simulink library "DQN_Machines"  (R2023b)
settings: Solver=VariableStepAuto  StartTime=0.0  StopTime=10.0  RelTol=1e-3
undefined symbols (not defined in the file): DiscIntNeverNeededParam, N, SM, Ts
libraries: spsabctodq0Lib x2, spsdq0toabcLib x2
(part 4 of 5)

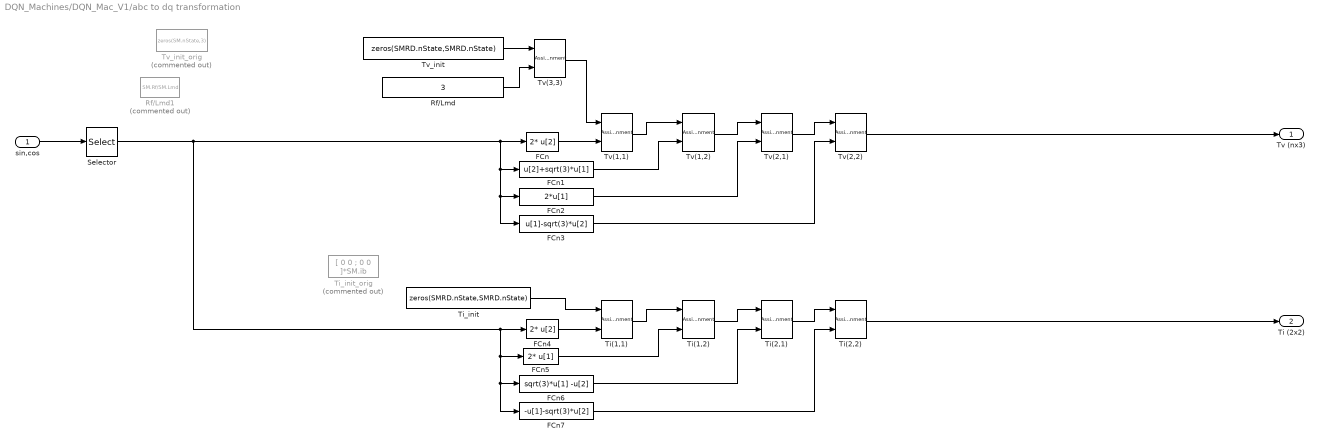
== system DQN_Machines/DQN_Mac_V1/abc to dq transformation ==
  sin,cos : Inport
  FCn : Fcn  Expr=2* u[2]  SampleTime=Ts
  FCn1 : Fcn  Expr=u[2]+sqrt(3)*u[1]  SampleTime=Ts
  FCn2 : Fcn  Expr=2*u[1]  SampleTime=Ts
  FCn3 : Fcn  Expr=u[1]-sqrt(3)*u[2]  SampleTime=Ts
  FCn4 : Fcn  Expr=2* u[2]  SampleTime=Ts
  FCn5 : Fcn  Expr=2* u[1]  SampleTime=Ts
  FCn6 : Fcn  Expr=sqrt(3)*u[1] -u[2]  SampleTime=Ts
  FCn7 : Fcn  Expr=-u[1]-sqrt(3)*u[2]  SampleTime=Ts
  Rf/Lmd : Constant  Value=3
  Rf/Lmd1 : Constant  Commented=on  Value=SM.Rf/SM.Lmd
  Selector : Selector  InputPortWidth=2  IndexOptions=Index vector (dialog)  Indices=[1 2]  OutputSizes=1
  "Ti(1,1) " : Assignment  NumberOfDimensions=2  DiagnosticForDimensions=Warning  IndexOptions=Index vector (dialog),Index vector (dialog)  Indices=1,1  OutputSizes=1,1
  "Ti(1,2) " : Assignment  NumberOfDimensions=2  DiagnosticForDimensions=Warning  IndexOptions=Index vector (dialog),Index vector (dialog)  Indices=1,2  OutputSizes=1,1
  "Ti(2,1) " : Assignment  NumberOfDimensions=2  DiagnosticForDimensions=Warning  IndexOptions=Index vector (dialog),Index vector (dialog)  Indices=2,1  OutputSizes=1,1
  "Ti(2,2) " : Assignment  NumberOfDimensions=2  DiagnosticForDimensions=Warning  IndexOptions=Index vector (dialog),Index vector (dialog)  Indices=2,2  OutputSizes=1,1
  Ti_init : Constant  Value=zeros(SMRD.nState,SMRD.nState)
  Ti_init_orig : Constant  Commented=on  Value="[ 0  0 ;  0  0  ]*SM.ib"
  Tv(1,1) : Assignment  NumberOfDimensions=2  DiagnosticForDimensions=Warning  IndexOptions=Index vector (dialog),Index vector (dialog)  Indices=1,1  OutputSizes=1,1
  Tv(1,2) : Assignment  NumberOfDimensions=2  DiagnosticForDimensions=Warning  IndexOptions=Index vector (dialog),Index vector (dialog)  Indices=1,2  OutputSizes=1,1
  Tv(2,1) : Assignment  NumberOfDimensions=2  DiagnosticForDimensions=Warning  IndexOptions=Index vector (dialog),Index vector (dialog)  Indices=2,1  OutputSizes=1,1
  Tv(2,2) : Assignment  NumberOfDimensions=2  DiagnosticForDimensions=Warning  IndexOptions=Index vector (dialog),Index vector (dialog)  Indices=2,2  OutputSizes=1,1
  Tv(3,3) : Assignment  NumberOfDimensions=2  DiagnosticForDimensions=Warning  IndexOptions=Index vector (dialog),Index vector (dialog)  Indices=3,3  OutputSizes=1,1
  Tv_init : Constant  Value=zeros(SMRD.nState,SMRD.nState)
  Tv_init_orig : Constant  Commented=on  Value=zeros(SM.nState,3)
  Tv (nx3) : Outport  VectorParamsAs1DForOutWhenUnconnected=off
  Ti (2x2) : Outport  Port=2  VectorParamsAs1DForOutWhenUnconnected=off
  wires:
  Tv(3,3)/1 -> Tv(1,1)/1
  Rf/Lmd/1 -> Tv(3,3)/2
  Tv_init/1 -> Tv(3,3)/1
  FCn7/1 -> "Ti(2,2) "/2
  "Ti(2,1) "/1 -> "Ti(2,2) "/1
  "Ti(1,2) "/1 -> "Ti(2,1) "/1
  FCn6/1 -> "Ti(2,1) "/2
  FCn5/1 -> "Ti(1,2) "/2
  "Ti(1,1) "/1 -> "Ti(1,2) "/1
  FCn4/1 -> "Ti(1,1) "/2
  FCn3/1 -> Tv(2,2)/2
  Tv(2,1)/1 -> Tv(2,2)/1
  Tv(1,2)/1 -> Tv(2,1)/1
  FCn2/1 -> Tv(2,1)/2
  FCn1/1 -> Tv(1,2)/2
  Tv(1,1)/1 -> Tv(1,2)/1
  FCn/1 -> Tv(1,1)/2
  sin,cos/1 -> Selector/1
  Ti_init/1 -> "Ti(1,1) "/1
  Selector/1 -> FCn7/1, FCn6/1, FCn5/1, FCn4/1, FCn/1, FCn1/1, FCn2/1, FCn3/1
  Tv(2,2)/1 -> Tv (nx3)/1
  "Ti(2,2) "/1 -> Ti (2x2)/1

== system DQN_Machines/DQN_Mac_V1/sin,cos ==
  theta : Inport
  Elementary Math : Trigonometry
  Elementary Math1 : Trigonometry  Operator=cos
  Mux3 : Mux  Inputs=2
  sin,cos : Outport  InitialOutput=0  VectorParamsAs1DForOutWhenUnconnected=off
  wires:
  theta/1 -> Elementary Math/1, Elementary Math1/1
  Elementary Math/1 -> Mux3/1
  Elementary Math1/1 -> Mux3/2
  Mux3/1 -> sin,cos/1

== system DQN_Machines/#BACKUP/DQN_Mac_V1/Discretize BE or Tustin2 ==
  note: Implement discretized state-space model using Tustin or TBE method
      |
      | BE      -> SM.DSSmethod=1
      | Tustin  -> SM.DSSmethod=2
      |
      |
      | Tustin
      | ------
      | Ad = inv(I - Ts/2*A)*(I + Ts/2*A)
      | Bd = inv(I - Ts/2*A)*B
      | Cd = C*inv(I - Ts/2*A)*Ts
      | Dd = C*inv(I - Ts/2*A)*B*Ts/2  + D  =  Cd*B/2
      |
      | TBE
      | ---
      | Ad = inv(I - Ts*A)
      | Bd = inv(I - Ts*A)*B
      | Cd = C*inv(I - Ts*A)*Ts
      | Dd = C*inv(I - Ts*A)*B*Ts  + D  =  Cd*B
      |
      | I = eye(SM.nState,SM.nState)
  A : Inport
  B : Inport  Port=2
  C : Inport  Port=3
  I : Constant  Value=eye(SMRD.nState,SMRD.nState)
  Product{1..4} (4 alike) : Product  Multiplication=Matrix(*)  SaturateOnIntegerOverflow=on  OutDataTypeStr=Inherit: Same as first input
  Sum1 : Sum  Inputs=+-  SaturateOnIntegerOverflow=on
  Sum5 : Sum  SaturateOnIntegerOverflow=on
  "Tustin: 1/2 BE : 1.0" : Gain  Gain=0.5  SaturateOnIntegerOverflow=on  OutDataTypeStr=Inherit: Same as input  ParamDataTypeStr=Inherit: Same as input
  "Tustin: Ts/2 BE : Ts" : Gain  Gain=SMRD.Ts/2  SaturateOnIntegerOverflow=on  OutDataTypeStr=Inherit: Same as input  ParamDataTypeStr=Inherit: Same as input
  inversion : Product  Inputs=/  Multiplication=Matrix(*)  RndMeth=Zero
  wbase3 : Gain  Gain=Ts  SaturateOnIntegerOverflow=on  OutDataTypeStr=Inherit: Same as input  ParamDataTypeStr=Inherit: Same as input
  Ad : Outport  VectorParamsAs1DForOutWhenUnconnected=off
  Bd : Outport  Port=2  VectorParamsAs1DForOutWhenUnconnected=off
  Cd : Outport  Port=3  VectorParamsAs1DForOutWhenUnconnected=off
  Dd : Outport  Port=4  VectorParamsAs1DForOutWhenUnconnected=off
  inv(I_Ts/2*A) : Outport  Port=5  VectorParamsAs1DForOutWhenUnconnected=off
  wires:
  "Tustin: Ts/2 BE : Ts"/1 -> Sum1/2, Sum5/2
  Product4/1 -> Ad/1
  A/1 -> "Tustin: Ts/2 BE : Ts"/1
  I/1 -> Sum5/1, Sum1/1
  Sum1/1 -> inversion/1
  inversion/1 -> Product2/2, Product1/1, Product4/1, inv(I_Ts/2*A)/1
  Sum5/1 -> Product4/2
  Product1/1 -> Bd/1
  B/1 -> Product1/2, Product3/2
  C/1 -> Product2/1
  Product2/1 -> wbase3/1
  Product3/1 -> "Tustin: 1/2 BE : 1.0"/1
  "Tustin: 1/2 BE : 1.0"/1 -> Dd/1
  wbase3/1 -> Cd/1, Product3/1

== system DQN_Machines/#BACKUP/DQN_Mac_V1/Electromagnetic Torque2 ==
  note: Te computed from stator fluxes and currents
  note: Te=phids*Iqs - phiqs*Ids
  phiqd : Inport
  iqd : Inport  Port=2
  1-1 : Gain  Gain=[-1 1]
  Mult1 : Product  Inputs=**
  Selector1 : Selector  InputPortWidth=2  IndexOptions=Index vector (dialog)  Indices="[2  1]"  OutputSizes=1
  Sum2 : Sum  Inputs=1  SaturateOnIntegerOverflow=on
  Te : Outport  VectorParamsAs1DForOutWhenUnconnected=off
  wires:
  phiqd/1 -> Selector1/1
  Mult1/1 -> Sum2/1
  iqd/1 -> 1-1/1
  1-1/1 -> Mult1/2  "iqs -ids"
  Selector1/1 -> Mult1/1  "phids phiqs"
  Sum2/1 -> Te/1

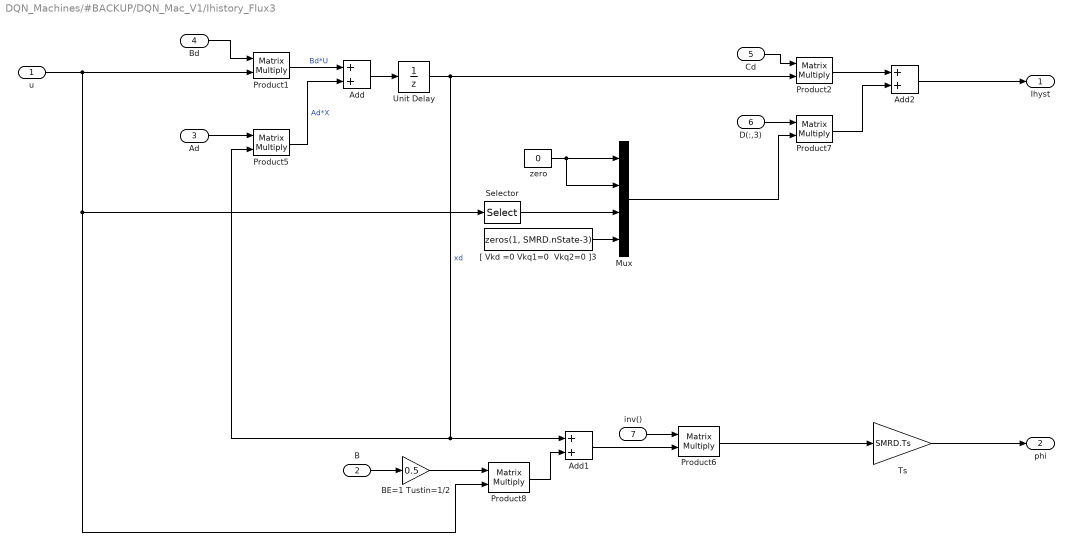
== system DQN_Machines/#BACKUP/DQN_Mac_V1/Ihistory_Flux3 ==
  u : Inport
  B : Inport  Port=2
  Ad : Inport  Port=3
  Bd : Inport  Port=4
  Cd : Inport  Port=5
  D(:,3) : Inport  Port=6
  inv() : Inport  Port=7
  Add : Sum
  Add1 : Sum
  Add2 : Sum
  BE=1 Tustin=1/2 : Gain  Gain=0.5
  Mux : Mux
  Product{1..2,5..8} (6 alike) : Product  Multiplication=Matrix(*)  SaturateOnIntegerOverflow=on  OutDataTypeStr=Inherit: Same as first input
  Selector : Selector  InputPortWidth=SMRD.nState  IndexOptions=Index vector (dialog)  Indices=[3]  OutputSizes=1
  Ts : Gain  Gain=SMRD.Ts  SaturateOnIntegerOverflow=on  OutDataTypeStr=Inherit: Same as input  ParamDataTypeStr=Inherit: Same as input
  Unit Delay : UnitDelay  InitialCondition=SMRD.phidq0(1:SMRD.nState)/SMRD.Ts  SampleTime=SMRD.Ts  HasFrameUpgradeWarning=on
  "[ Vkd =0 Vkq1=0  Vkq2=0 ]3" : Constant  Value=zeros(1, SMRD.nState-3)
  zero : Constant  Value=0
  Ihyst : Outport  VectorParamsAs1DForOutWhenUnconnected=off
  phi : Outport  Port=2  VectorParamsAs1DForOutWhenUnconnected=off
  wires:
  BE=1 Tustin=1/2/1 -> Product8/1
  u/1 -> Product1/2, Product8/2, Selector/1
  B/1 -> BE=1 Tustin=1/2/1
  inv()/1 -> Product6/1
  Cd/1 -> Product2/1
  Bd/1 -> Product1/1
  Ad/1 -> Product5/1
  Add1/1 -> Product6/2
  Product8/1 -> Add1/2
  Product6/1 -> Ts/1
  Product5/1 -> Add/2  "Ad*X"
  Unit Delay/1 -> Product5/2, Add1/1, Product2/2  "xd"
  Add/1 -> Unit Delay/1
  Product1/1 -> Add/1  "Bd*U"
  Ts/1 -> phi/1
  Product2/1 -> Add2/1
  Add2/1 -> Ihyst/1
  Mux/1 -> Product7/2
  D(:,3)/1 -> Product7/1
  "[ Vkd =0 Vkq1=0  Vkq2=0 ]3"/1 -> Mux/4
  zero/1 -> Mux/2, Mux/1
  Selector/1 -> Mux/3
  Product7/1 -> Add2/2

== system DQN_Machines/#BACKUP/DQN_Mac_V1/Matrix W3 ==
  wr : Inport
  Gain1 : Gain  Gain=-1  SaturateOnIntegerOverflow=on  OutDataTypeStr=Inherit: Same as input  ParamDataTypeStr=Inherit: Same as input
  Gain2 : Gain  Gain=-1  SaturateOnIntegerOverflow=on  OutDataTypeStr=Inherit: Same as input  ParamDataTypeStr=Inherit: Same as input
  W(1,2)=wr : Assignment  NumberOfDimensions=2  IndexOptions=Index vector (dialog),Index vector (dialog)  Indices=1,2  OutputSizes=1,1
  W(2,1)=-wr : Assignment  NumberOfDimensions=2  IndexOptions=Index vector (dialog),Index vector (dialog)  Indices=2,1  OutputSizes=1,1
  u1 : Constant  Value=zeros(SMRD.nState,SMRD.nState)
  "[W]" : Outport  VectorParamsAs1DForOutWhenUnconnected=off
  wires:
  u1/1 -> W(1,2)=wr/1
  Gain1/1 -> W(2,1)=-wr/2
  W(1,2)=wr/1 -> W(2,1)=-wr/1
  wr/1 -> W(1,2)=wr/2, Gain1/1
  W(2,1)=-wr/1 -> Gain2/1
  Gain2/1 -> "[W]"/1

== system DQN_Machines/#BACKUP/DQN_Mac_V1/Mechanical model ==
  note: *
  note: Computation of Rotor angle dthetae uses Forward Euler
      | integrator to ensure better accuracy and initialisation.
  note: *
  Te : Inport  PortDimensions=1
  Pm : Inport  Port=2
  1 ----- 2H : Gain  Gain=1/(2*SMRD.H)  SaturateOnIntegerOverflow=on  OutDataTypeStr=Inherit: Same as input  ParamDataTypeStr=Inherit: Same as input
  1_Pb : Gain  Gain=1/SMRD.Pb  SaturateOnIntegerOverflow=on  OutDataTypeStr=Inherit: Same as input  ParamDataTypeStr=Inherit: Same as input
  Delay Prediction : Subsystem
  Digital Clock : DigitalClock  SampleTime=Ts
  F : Gain  Gain=SMRD.F  SaturateOnIntegerOverflow=on  OutDataTypeStr=Inherit: Same as input  ParamDataTypeStr=Inherit: Same as input
  Mux1 : Mux  Inputs=2
  Rate Transition1 : RateTransition  Deterministic=off  OutPortSampleTime=Ts
  Rotor angle dthetae : DiscreteIntegrator  InitialCondition=SMRD.tho  SampleTime=SMRD.Ts  ICPrevOutput=DiscIntNeverNeededParam  ICPrevScaledInput=DiscIntNeverNeededParam
  Rotor speed deviation (dw) : DiscreteIntegrator  IntegratorMethod=Integration: Trapezoidal  InitialCondition=SMRD.dwo  SampleTime=SMRD.Ts  ICPrevOutput=DiscIntNeverNeededParam  ICPrevScaledInput=DiscIntNeverNeededParam
  Sum : Sum  InputSameDT=on  SaturateOnIntegerOverflow=on  OutDataTypeStr=Inherit: Same as first input
  Sum2 : Sum  Inputs=+--  InputSameDT=on  SaturateOnIntegerOverflow=on  OutDataTypeStr=Inherit: Same as first input
  Sum3 : Sum  InputSameDT=on  SaturateOnIntegerOverflow=on  OutDataTypeStr=Inherit: Same as first input
  div : Fcn  Expr=u[2]/u[1]
      mask Display: disp('/')
  nominal speed : Constant
  we base : Gain  Gain=SMRD.wn  SaturateOnIntegerOverflow=on  OutDataTypeStr=Inherit: Same as input  ParamDataTypeStr=Inherit: Same as input
  web2 : Gain  Gain=SMRD.wn  SaturateOnIntegerOverflow=on  OutDataTypeStr=Inherit: Same as input  ParamDataTypeStr=Inherit: Same as input
  dtheta_e : Outport  InitialOutput=0  VectorParamsAs1DForOutWhenUnconnected=off
  we : Outport  Port=2  InitialOutput=0  VectorParamsAs1DForOutWhenUnconnected=off
  theta_e : Outport  Port=3  InitialOutput=0  VectorParamsAs1DForOutWhenUnconnected=off
  wires:
  Delay Prediction/1(dw) -> we base/1, Sum/2  "dw"
  Rate Transition1/1 -> 1_Pb/1
  Rotor angle dthetae/1 -> Sum3/1, dtheta_e/1  "d_theta (rad)"
  web2/1 -> Sum3/2
  Digital Clock/1 -> web2/1
  we base/1 -> Rotor angle dthetae/1
  Rotor speed deviation (dw)/1 -> Delay Prediction/1(in)  "dw"
  nominal speed/1 -> Sum/1
  1 ----- 2H/1 -> Rotor speed deviation (dw)/1
  div/1 -> Sum2/1
  Te/1 -> Sum2/2  "Te"
  Mux1/1 -> div/1
  Pm/1 -> Rate Transition1/1  "Pm"
  1_Pb/1 -> Mux1/2
  F/1 -> Sum2/3
  Sum2/1 -> 1 ----- 2H/1
  Sum/1 -> F/1, we/1, Mux1/1  "n"
  Sum3/1 -> theta_e/1

== system DQN_Machines/#BACKUP/DQN_Mac_V1_old/Electromagnetic Torque1 ==
  note: Te computed from stator fluxes and currents
  note: Te=phids*Iqs - phiqs*Ids
  phiqd : Inport
  iqd : Inport  Port=2
  1-1 : Gain  Gain=[-1 1]
  Mult1 : Product  Inputs=**
  Selector1 : Selector  InputPortWidth=2  IndexOptions=Index vector (dialog)  Indices="[2  1]"  OutputSizes=1
  Sum2 : Sum  Inputs=1  SaturateOnIntegerOverflow=on
  Te : Outport  VectorParamsAs1DForOutWhenUnconnected=off
  wires:
  phiqd/1 -> Selector1/1
  Mult1/1 -> Sum2/1
  iqd/1 -> 1-1/1
  1-1/1 -> Mult1/2  "iqs -ids"
  Selector1/1 -> Mult1/1  "phids phiqs"
  Sum2/1 -> Te/1

== system DQN_Machines/#BACKUP/DQN_Mac_V1_old/Ihistory_Flux ==
  A : Inport
  u_dq : Inport  Port=2
  Add2 : Sum
  Add3 : Sum
  BE=1 Tustin=1/2 : Gain  Gain=0.5
  I : Constant  Value=eye(SMRD.nState,SMRD.nState)
  Product{4..5,7..8} (4 alike) : Product  Multiplication=Matrix(*)  SaturateOnIntegerOverflow=on  OutDataTypeStr=Inherit: Same as first input
  Sum1 : Sum  Inputs=+-  SaturateOnIntegerOverflow=on
  Sum5 : Sum  SaturateOnIntegerOverflow=on
  Ts : Gain  Gain=SMRD.Ts  SaturateOnIntegerOverflow=on  OutDataTypeStr=Inherit: Same as input  ParamDataTypeStr=Inherit: Same as input
  "Tustin: Ts/2 BE : Ts" : Gain  Gain=SMRD.Ts/2  SaturateOnIntegerOverflow=on  OutDataTypeStr=Inherit: Same as input  ParamDataTypeStr=Inherit: Same as input
  Unit Delay2 : UnitDelay  InitialCondition=SMRD.phidq0/SMRD.Ts  SampleTime=SMRD.Ts  HasFrameUpgradeWarning=on
  inversion : Product  Inputs=/  Multiplication=Matrix(*)  RndMeth=Zero
  phi : Outport  VectorParamsAs1DForOutWhenUnconnected=off
  wires:
  Unit Delay2/1 -> Add3/1, Product4/2  "xd"
  Add2/1 -> Unit Delay2/1
  Product4/1 -> Add2/2  "Ad*X"
  Product5/1 -> Product4/1
  Product7/1 -> Ts/1
  Add3/1 -> Product7/2
  inversion/1 -> Product7/1, Product8/1, Product5/1
  Ts/1 -> phi/1
  u_dq/1 -> Product8/2, BE=1 Tustin=1/2/1
  Sum1/1 -> inversion/1
  Sum5/1 -> Product5/2
  I/1 -> Sum5/1, Sum1/1
  A/1 -> "Tustin: Ts/2 BE : Ts"/1
  "Tustin: Ts/2 BE : Ts"/1 -> Sum5/2, Sum1/2
  BE=1 Tustin=1/2/1 -> Add3/2
  Product8/1 -> Add2/1

== system DQN_Machines/#BACKUP/DQN_Mac_V1_old/Matrix W3 ==
  wr : Inport
  Gain1 : Gain  Gain=-1  SaturateOnIntegerOverflow=on  OutDataTypeStr=Inherit: Same as input  ParamDataTypeStr=Inherit: Same as input
  W(1,2)=wr : Assignment  NumberOfDimensions=2  IndexOptions=Index vector (dialog),Index vector (dialog)  Indices=1,2  OutputSizes=1,1
  W(2,1)=-wr : Assignment  NumberOfDimensions=2  IndexOptions=Index vector (dialog),Index vector (dialog)  Indices=2,1  OutputSizes=1,1
  u1 : Constant  Value=zeros(SMRD.nState,SMRD.nState)
  "[W]" : Outport  VectorParamsAs1DForOutWhenUnconnected=off
  wires:
  u1/1 -> W(1,2)=wr/1
  wr/1 -> W(2,1)=-wr/2, W(1,2)=wr/2
  W(1,2)=wr/1 -> Gain1/1
  W(2,1)=-wr/1 -> "[W]"/1
  Gain1/1 -> W(2,1)=-wr/1

== system DQN_Machines/#BACKUP/DQN_Mac_V1_old/Mechanical model ==
  note: *
  note: Computation of Rotor angle dthetae uses Forward Euler
      | integrator to ensure better accuracy and initialisation.
  note: *
  Te : Inport  PortDimensions=1
  Pm : Inport  Port=2
  1 ----- 2H : Gain  Gain=1/(2*SMRD.H)  SaturateOnIntegerOverflow=on  OutDataTypeStr=Inherit: Same as input  ParamDataTypeStr=Inherit: Same as input
  1_Pb : Gain  Gain=1/SMRD.Pb  SaturateOnIntegerOverflow=on  OutDataTypeStr=Inherit: Same as input  ParamDataTypeStr=Inherit: Same as input
  Delay Prediction : Subsystem
  Digital Clock : DigitalClock  SampleTime=SMRD.Ts
  F : Gain  Gain=SMRD.F  SaturateOnIntegerOverflow=on  OutDataTypeStr=Inherit: Same as input  ParamDataTypeStr=Inherit: Same as input
  Mux1 : Mux  Inputs=2
  Rate Transition1 : RateTransition  Commented=on  Deterministic=off  OutPortSampleTime=SMRD.Ts
  Rotor angle dthetae : DiscreteIntegrator  InitialCondition=SMRD.tho  SampleTime=SMRD.Ts  ICPrevOutput=DiscIntNeverNeededParam  ICPrevScaledInput=DiscIntNeverNeededParam
  Rotor speed deviation (dw) : DiscreteIntegrator  IntegratorMethod=Integration: Trapezoidal  InitialCondition=SMRD.dwo  SampleTime=SMRD.Ts  ICPrevOutput=DiscIntNeverNeededParam  ICPrevScaledInput=DiscIntNeverNeededParam
  Sum : Sum  InputSameDT=on  SaturateOnIntegerOverflow=on  OutDataTypeStr=Inherit: Same as first input
  Sum2 : Sum  Inputs=+--  InputSameDT=on  SaturateOnIntegerOverflow=on  OutDataTypeStr=Inherit: Same as first input
  Sum3 : Sum  InputSameDT=on  SaturateOnIntegerOverflow=on  OutDataTypeStr=Inherit: Same as first input
  div : Fcn  Expr=u[2]/u[1]
      mask Display: disp('/')
  nominal speed : Constant
  we base : Gain  Gain=SMRD.web  SaturateOnIntegerOverflow=on  OutDataTypeStr=Inherit: Same as input  ParamDataTypeStr=Inherit: Same as input
  web2 : Gain  Gain=SMRD.web  SaturateOnIntegerOverflow=on  OutDataTypeStr=Inherit: Same as input  ParamDataTypeStr=Inherit: Same as input
  we : Outport
  theta_e : Outport  Port=2  InitialOutput=0  VectorParamsAs1DForOutWhenUnconnected=off
  dtheta_e : Outport  Port=3  InitialOutput=0  VectorParamsAs1DForOutWhenUnconnected=off
  wires:
  Delay Prediction/1(dw) -> we base/1, Sum/2  "dw"
  Rotor angle dthetae/1 -> dtheta_e/1, Sum3/1  "d_theta (rad)"
  web2/1 -> Sum3/2
  Digital Clock/1 -> web2/1
  we base/1 -> Rotor angle dthetae/1
  Rotor speed deviation (dw)/1 -> Delay Prediction/1(in)  "dw"
  nominal speed/1 -> Sum/1
  1 ----- 2H/1 -> Rotor speed deviation (dw)/1
  div/1 -> Sum2/1
  Te/1 -> Sum2/2  "Te"
  Mux1/1 -> div/1
  Pm/1 -> 1_Pb/1  "Pm"
  1_Pb/1 -> Mux1/2
  F/1 -> Sum2/3
  Sum2/1 -> 1 ----- 2H/1
  Sum/1 -> F/1, we/1, Mux1/1  "n"
  Sum3/1 -> theta_e/1

== system DQN_Machines/#BACKUP/DQN_Mac_V1_old/mac_pnz2dq_conv ==
  In1 : Inport
  Complex to Real-Imag : ComplexToRealImag
  Mux : Mux  Inputs=2
  Sel4 : Selector  NumberOfDimensions=2  InputPortWidth=3  IndexOptions=Index vector (dialog),Index vector (dialog)  Indices=1,2  OutputSizes=1
  Out4 : Outport
  wires:
  Complex to Real-Imag/1 -> Mux/1
  Sel4/1 -> Complex to Real-Imag/1
  In1/1 -> Sel4/1
  Mux/1 -> Out4/1
  Complex to Real-Imag/2 -> Mux/2

== system DQN_Machines/#BACKUP/DQN_Mac_V2/Discretize BE or Tustin2 ==
  note: Implement discretized state-space model using Tustin or TBE method
      |
      | BE      -> SM.DSSmethod=1
      | Tustin  -> SM.DSSmethod=2
      |
      |
      | Tustin
      | ------
      | Ad = inv(I - Ts/2*A)*(I + Ts/2*A)
      | Bd = inv(I - Ts/2*A)*B
      | Cd = C*inv(I - Ts/2*A)*Ts
      | Dd = C*inv(I - Ts/2*A)*B*Ts/2  + D  =  Cd*B/2
      |
      | TBE
      | ---
      | Ad = inv(I - Ts*A)
      | Bd = inv(I - Ts*A)*B
      | Cd = C*inv(I - Ts*A)*Ts
      | Dd = C*inv(I - Ts*A)*B*Ts  + D  =  Cd*B
      |
      | I = eye(SM.nState,SM.nState)
  A : Inport
  B : Inport  Port=2
  C : Inport  Port=3
  I : Constant  Value=eye(SMRD.nState,SMRD.nState)
  Product{1..4} (4 alike) : Product  Multiplication=Matrix(*)  SaturateOnIntegerOverflow=on  OutDataTypeStr=Inherit: Same as first input
  Sum1 : Sum  Inputs=+-  SaturateOnIntegerOverflow=on
  Sum5 : Sum  SaturateOnIntegerOverflow=on
  "Tustin: 1/2 BE : 1.0" : Gain  Gain=0.5  SaturateOnIntegerOverflow=on  OutDataTypeStr=Inherit: Same as input  ParamDataTypeStr=Inherit: Same as input
  "Tustin: Ts/2 BE : Ts" : Gain  Gain=SMRD.Ts/2  SaturateOnIntegerOverflow=on  OutDataTypeStr=Inherit: Same as input  ParamDataTypeStr=Inherit: Same as input
  inversion : Product  Inputs=/  Multiplication=Matrix(*)  RndMeth=Zero
  wbase3 : Gain  Gain=Ts  SaturateOnIntegerOverflow=on  OutDataTypeStr=Inherit: Same as input  ParamDataTypeStr=Inherit: Same as input
  Ad : Outport  VectorParamsAs1DForOutWhenUnconnected=off
  Bd : Outport  Port=2  VectorParamsAs1DForOutWhenUnconnected=off
  Cd : Outport  Port=3  VectorParamsAs1DForOutWhenUnconnected=off
  Dd : Outport  Port=4  VectorParamsAs1DForOutWhenUnconnected=off
  inv(I_Ts/2*A) : Outport  Port=5  VectorParamsAs1DForOutWhenUnconnected=off
  wires:
  wbase3/1 -> Product3/1, Cd/1
  "Tustin: 1/2 BE : 1.0"/1 -> Dd/1
  Product3/1 -> "Tustin: 1/2 BE : 1.0"/1
  Product2/1 -> wbase3/1
  C/1 -> Product2/1
  B/1 -> Product3/2, Product1/2
  Product1/1 -> Bd/1
  Sum5/1 -> Product4/2
  inversion/1 -> inv(I_Ts/2*A)/1, Product4/1, Product1/1, Product2/2
  Sum1/1 -> inversion/1
  I/1 -> Sum1/1, Sum5/1
  A/1 -> "Tustin: Ts/2 BE : Ts"/1
  Product4/1 -> Ad/1
  "Tustin: Ts/2 BE : Ts"/1 -> Sum5/2, Sum1/2

== system DQN_Machines/#BACKUP/DQN_Mac_V2/Electromagnetic Torque2 ==
  note: Te=phids*Iqs - phiqs*Ids
  note: Te computed from stator fluxes and currents
  phiqd : Inport
  iqd : Inport  Port=2
  1-1 : Gain  Gain=[-1 1]
  Mult1 : Product  Inputs=**
  Selector1 : Selector  InputPortWidth=2  IndexOptions=Index vector (dialog)  Indices="[2  1]"  OutputSizes=1
  Sum2 : Sum  Inputs=1  SaturateOnIntegerOverflow=on
  Te : Outport  VectorParamsAs1DForOutWhenUnconnected=off
  wires:
  Sum2/1 -> Te/1
  Selector1/1 -> Mult1/1  "phids phiqs"
  1-1/1 -> Mult1/2  "iqs -ids"
  iqd/1 -> 1-1/1
  Mult1/1 -> Sum2/1
  phiqd/1 -> Selector1/1

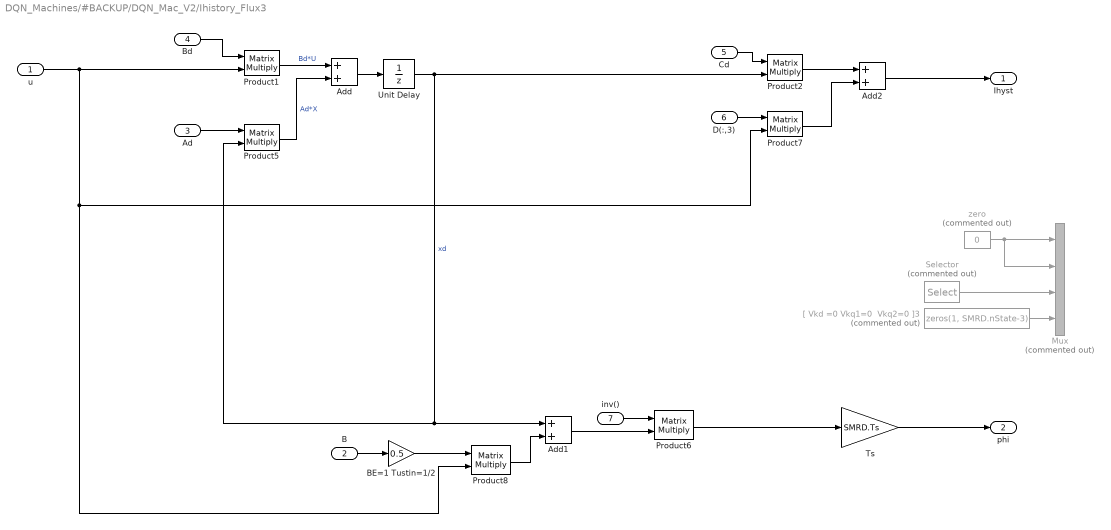
== system DQN_Machines/#BACKUP/DQN_Mac_V2/Ihistory_Flux3 ==
  u : Inport
  B : Inport  Port=2
  Ad : Inport  Port=3
  Bd : Inport  Port=4
  Cd : Inport  Port=5
  D(:,3) : Inport  Port=6
  inv() : Inport  Port=7
  Add : Sum
  Add1 : Sum
  Add2 : Sum
  BE=1 Tustin=1/2 : Gain  Gain=0.5
  Mux : Mux  Commented=on
  Product{1..2,5..8} (6 alike) : Product  Multiplication=Matrix(*)  SaturateOnIntegerOverflow=on  OutDataTypeStr=Inherit: Same as first input
  Selector : Selector  Commented=on  InputPortWidth=SMRD.nState  IndexOptions=Index vector (dialog)  Indices=[3]  OutputSizes=1
  Ts : Gain  Gain=SMRD.Ts  SaturateOnIntegerOverflow=on  OutDataTypeStr=Inherit: Same as input  ParamDataTypeStr=Inherit: Same as input
  Unit Delay : UnitDelay  InitialCondition=SMRD.phidq0(1:SMRD.nState)/SMRD.Ts  SampleTime=SMRD.Ts  HasFrameUpgradeWarning=on
  "[ Vkd =0 Vkq1=0  Vkq2=0 ]3" : Constant  Commented=on  Value=zeros(1, SMRD.nState-3)
  zero : Constant  Commented=on  Value=0
  Ihyst : Outport  VectorParamsAs1DForOutWhenUnconnected=off
  phi : Outport  Port=2  VectorParamsAs1DForOutWhenUnconnected=off
  wires:
  Product7/1 -> Add2/2
  D(:,3)/1 -> Product7/1
  u/1 -> Product7/2, Product8/2, Product1/2
  Add2/1 -> Ihyst/1
  Product2/1 -> Add2/1
  Ts/1 -> phi/1
  Product1/1 -> Add/1  "Bd*U"
  Add/1 -> Unit Delay/1
  Unit Delay/1 -> Product2/2, Add1/1, Product5/2  "xd"
  Product5/1 -> Add/2  "Ad*X"
  Product6/1 -> Ts/1
  Product8/1 -> Add1/2
  Add1/1 -> Product6/2
  Ad/1 -> Product5/1
  Bd/1 -> Product1/1
  Cd/1 -> Product2/1
  inv()/1 -> Product6/1
  B/1 -> BE=1 Tustin=1/2/1
  BE=1 Tustin=1/2/1 -> Product8/1
  "[ Vkd =0 Vkq1=0  Vkq2=0 ]3"/1 -> Mux/4
  zero/1 -> Mux/1, Mux/2
  Selector/1 -> Mux/3

== system DQN_Machines/#BACKUP/DQN_Mac_V2/Matrix W3 ==
  wr : Inport
  Gain1 : Gain  Gain=-1  SaturateOnIntegerOverflow=on  OutDataTypeStr=Inherit: Same as input  ParamDataTypeStr=Inherit: Same as input
  Gain2 : Gain  Gain=-1  SaturateOnIntegerOverflow=on  OutDataTypeStr=Inherit: Same as input  ParamDataTypeStr=Inherit: Same as input
  W(1,2)=wr : Assignment  NumberOfDimensions=2  IndexOptions=Index vector (dialog),Index vector (dialog)  Indices=1,2  OutputSizes=1,1
  W(2,1)=-wr : Assignment  NumberOfDimensions=2  IndexOptions=Index vector (dialog),Index vector (dialog)  Indices=2,1  OutputSizes=1,1
  u1 : Constant  Value=zeros(SMRD.nState,SMRD.nState)
  "[W]" : Outport  VectorParamsAs1DForOutWhenUnconnected=off
  wires:
  Gain2/1 -> "[W]"/1
  W(2,1)=-wr/1 -> Gain2/1
  wr/1 -> Gain1/1, W(1,2)=wr/2
  W(1,2)=wr/1 -> W(2,1)=-wr/1
  Gain1/1 -> W(2,1)=-wr/2
  u1/1 -> W(1,2)=wr/1

== system DQN_Machines/#BACKUP/DQN_Mac_V2/Mechanical model ==
  note: *
  note: Computation of Rotor angle dthetae uses Forward Euler
      | integrator to ensure better accuracy and initialisation.
  note: *
  Te : Inport  PortDimensions=1
  Pm : Inport  Port=2
  1 ----- 2H : Gain  Gain=1/(2*SMRD.H)  SaturateOnIntegerOverflow=on  OutDataTypeStr=Inherit: Same as input  ParamDataTypeStr=Inherit: Same as input
  1_Pb : Gain  Gain=1/SMRD.Pb  SaturateOnIntegerOverflow=on  OutDataTypeStr=Inherit: Same as input  ParamDataTypeStr=Inherit: Same as input
  Delay Prediction : Subsystem
  Digital Clock : DigitalClock  SampleTime=Ts
  F : Gain  Gain=SMRD.F  SaturateOnIntegerOverflow=on  OutDataTypeStr=Inherit: Same as input  ParamDataTypeStr=Inherit: Same as input
  Mux1 : Mux  Inputs=2
  Rate Transition1 : RateTransition  Deterministic=off  OutPortSampleTime=Ts
  Rotor angle dthetae : DiscreteIntegrator  InitialCondition=SMRD.tho  SampleTime=SMRD.Ts  ICPrevOutput=DiscIntNeverNeededParam  ICPrevScaledInput=DiscIntNeverNeededParam
  Rotor speed deviation (dw) : DiscreteIntegrator  IntegratorMethod=Integration: Trapezoidal  InitialCondition=SMRD.dwo  SampleTime=SMRD.Ts  ICPrevOutput=DiscIntNeverNeededParam  ICPrevScaledInput=DiscIntNeverNeededParam
  Sum : Sum  InputSameDT=on  SaturateOnIntegerOverflow=on  OutDataTypeStr=Inherit: Same as first input
  Sum2 : Sum  Inputs=+--  InputSameDT=on  SaturateOnIntegerOverflow=on  OutDataTypeStr=Inherit: Same as first input
  Sum3 : Sum  InputSameDT=on  SaturateOnIntegerOverflow=on  OutDataTypeStr=Inherit: Same as first input
  div : Fcn  Expr=u[2]/u[1]
      mask Display: disp('/')
  nominal speed : Constant
  we base : Gain  Gain=SMRD.wn  SaturateOnIntegerOverflow=on  OutDataTypeStr=Inherit: Same as input  ParamDataTypeStr=Inherit: Same as input
  web2 : Gain  Gain=SMRD.wn  SaturateOnIntegerOverflow=on  OutDataTypeStr=Inherit: Same as input  ParamDataTypeStr=Inherit: Same as input
  dtheta_e : Outport  InitialOutput=0  VectorParamsAs1DForOutWhenUnconnected=off
  we : Outport  Port=2  InitialOutput=0  VectorParamsAs1DForOutWhenUnconnected=off
  theta_e : Outport  Port=3  InitialOutput=0  VectorParamsAs1DForOutWhenUnconnected=off
  wires:
  Sum3/1 -> theta_e/1
  Sum/1 -> Mux1/1, we/1, F/1  "n"
  Sum2/1 -> 1 ----- 2H/1
  F/1 -> Sum2/3
  1_Pb/1 -> Mux1/2
  Pm/1 -> Rate Transition1/1  "Pm"
  Mux1/1 -> div/1
  Te/1 -> Sum2/2  "Te"
  div/1 -> Sum2/1
  1 ----- 2H/1 -> Rotor speed deviation (dw)/1
  nominal speed/1 -> Sum/1
  Rotor speed deviation (dw)/1 -> Delay Prediction/1(in)  "dw"
  we base/1 -> Rotor angle dthetae/1
  Digital Clock/1 -> web2/1
  web2/1 -> Sum3/2
  Rotor angle dthetae/1 -> dtheta_e/1, Sum3/1  "d_theta (rad)"
  Rate Transition1/1 -> 1_Pb/1
  Delay Prediction/1(dw) -> Sum/2, we base/1  "dw"

== system DQN_Machines/#BACKUP/DQN_Mac_V2_untested/Discretize BE or Tustin2 ==
  note: Implement discretized state-space model using Tustin or TBE method
      |
      | BE      -> SM.DSSmethod=1
      | Tustin  -> SM.DSSmethod=2
      |
      |
      | Tustin
      | ------
      | Ad = inv(I - Ts/2*A)*(I + Ts/2*A)
      | Bd = inv(I - Ts/2*A)*B
      | Cd = C*inv(I - Ts/2*A)*Ts
      | Dd = C*inv(I - Ts/2*A)*B*Ts/2  + D  =  Cd*B/2
      |
      | TBE
      | ---
      | Ad = inv(I - Ts*A)
      | Bd = inv(I - Ts*A)*B
      | Cd = C*inv(I - Ts*A)*Ts
      | Dd = C*inv(I - Ts*A)*B*Ts  + D  =  Cd*B
      |
      | I = eye(SM.nState,SM.nState)
  A : Inport
  B : Inport  Port=2
  C : Inport  Port=3
  I : Constant  Value=eye(SMRD.nState,SMRD.nState)
  Product{1..4} (4 alike) : Product  Multiplication=Matrix(*)  SaturateOnIntegerOverflow=on  OutDataTypeStr=Inherit: Same as first input
  Sum1 : Sum  Inputs=+-  SaturateOnIntegerOverflow=on
  Sum5 : Sum  SaturateOnIntegerOverflow=on
  "Tustin: 1/2 BE : 1.0" : Gain  Gain=0.5  SaturateOnIntegerOverflow=on  OutDataTypeStr=Inherit: Same as input  ParamDataTypeStr=Inherit: Same as input
  "Tustin: Ts/2 BE : Ts" : Gain  Gain=SMRD.Ts/2  SaturateOnIntegerOverflow=on  OutDataTypeStr=Inherit: Same as input  ParamDataTypeStr=Inherit: Same as input
  inversion : Product  Inputs=/  Multiplication=Matrix(*)  RndMeth=Zero
  wbase3 : Gain  Gain=Ts  SaturateOnIntegerOverflow=on  OutDataTypeStr=Inherit: Same as input  ParamDataTypeStr=Inherit: Same as input
  Ad : Outport  VectorParamsAs1DForOutWhenUnconnected=off
  Bd : Outport  Port=2  VectorParamsAs1DForOutWhenUnconnected=off
  Cd : Outport  Port=3  VectorParamsAs1DForOutWhenUnconnected=off
  Dd : Outport  Port=4  VectorParamsAs1DForOutWhenUnconnected=off
  inv(I_Ts/2*A) : Outport  Port=5  VectorParamsAs1DForOutWhenUnconnected=off
  wires:
  "Tustin: Ts/2 BE : Ts"/1 -> Sum1/2, Sum5/2
  Product4/1 -> Ad/1
  A/1 -> "Tustin: Ts/2 BE : Ts"/1
  I/1 -> Sum5/1, Sum1/1
  Sum1/1 -> inversion/1
  inversion/1 -> Product2/2, Product1/1, Product4/1, inv(I_Ts/2*A)/1
  Sum5/1 -> Product4/2
  Product1/1 -> Bd/1
  B/1 -> Product1/2, Product3/2
  C/1 -> Product2/1
  Product2/1 -> wbase3/1
  Product3/1 -> "Tustin: 1/2 BE : 1.0"/1
  "Tustin: 1/2 BE : 1.0"/1 -> Dd/1
  wbase3/1 -> Cd/1, Product3/1

== system DQN_Machines/#BACKUP/DQN_Mac_V2_untested/Electromagnetic Torque2 ==
  note: Te computed from stator fluxes and currents
  note: Te=phids*Iqs - phiqs*Ids
  phiqd : Inport
  iqd : Inport  Port=2
  1-1 : Gain  Gain=[-1 1]
  Mult1 : Product  Inputs=**
  Selector1 : Selector  InputPortWidth=2  IndexOptions=Index vector (dialog)  Indices="[2  1]"  OutputSizes=1
  Sum2 : Sum  Inputs=1  SaturateOnIntegerOverflow=on
  Te : Outport  VectorParamsAs1DForOutWhenUnconnected=off
  wires:
  phiqd/1 -> Selector1/1
  Mult1/1 -> Sum2/1
  iqd/1 -> 1-1/1
  1-1/1 -> Mult1/2  "iqs -ids"
  Selector1/1 -> Mult1/1  "phids phiqs"
  Sum2/1 -> Te/1

== system DQN_Machines/#BACKUP/DQN_Mac_V2_untested/Ihistory_Flux3 ==
  u : Inport
  B : Inport  Port=2
  Ad : Inport  Port=3
  Bd : Inport  Port=4
  Cd : Inport  Port=5
  D(:,3) : Inport  Port=6
  inv() : Inport  Port=7
  Add : Sum
  Add1 : Sum
  Add2 : Sum
  BE=1 Tustin=1/2 : Gain  Gain=0.5
  Mux : Mux  Commented=on
  Product{1..2,5..8} (6 alike) : Product  Multiplication=Matrix(*)  SaturateOnIntegerOverflow=on  OutDataTypeStr=Inherit: Same as first input
  Selector : Selector  Commented=on  InputPortWidth=SMRD.nState  IndexOptions=Index vector (dialog)  Indices=[3]  OutputSizes=1
  Ts : Gain  Gain=SMRD.Ts  SaturateOnIntegerOverflow=on  OutDataTypeStr=Inherit: Same as input  ParamDataTypeStr=Inherit: Same as input
  Unit Delay : UnitDelay  InitialCondition=SMRD.phidq0(1:SMRD.nState)/SMRD.Ts  SampleTime=SMRD.Ts  HasFrameUpgradeWarning=on
  "[ Vkd =0 Vkq1=0  Vkq2=0 ]3" : Constant  Commented=on  Value=zeros(1, SMRD.nState-3)
  zero : Constant  Commented=on  Value=0
  Ihyst : Outport  VectorParamsAs1DForOutWhenUnconnected=off
  phi : Outport  Port=2  VectorParamsAs1DForOutWhenUnconnected=off
  wires:
  Selector/1 -> Mux/3
  zero/1 -> Mux/2, Mux/1
  "[ Vkd =0 Vkq1=0  Vkq2=0 ]3"/1 -> Mux/4
  BE=1 Tustin=1/2/1 -> Product8/1
  B/1 -> BE=1 Tustin=1/2/1
  inv()/1 -> Product6/1
  Cd/1 -> Product2/1
  Bd/1 -> Product1/1
  Ad/1 -> Product5/1
  Add1/1 -> Product6/2
  Product8/1 -> Add1/2
  Product6/1 -> Ts/1
  Product5/1 -> Add/2  "Ad*X"
  Unit Delay/1 -> Add1/1, Product5/2, Product2/2  "xd"
  Add/1 -> Unit Delay/1
  Product1/1 -> Add/1  "Bd*U"
  Ts/1 -> phi/1
  Product2/1 -> Add2/1
  Add2/1 -> Ihyst/1
  u/1 -> Product1/2, Product8/2, Product7/2
  D(:,3)/1 -> Product7/1
  Product7/1 -> Add2/2

== system DQN_Machines/#BACKUP/DQN_Mac_V2_untested/Matrix W3 ==
  wr : Inport
  Gain1 : Gain  Gain=-1  SaturateOnIntegerOverflow=on  OutDataTypeStr=Inherit: Same as input  ParamDataTypeStr=Inherit: Same as input
  Gain2 : Gain  Gain=-1  SaturateOnIntegerOverflow=on  OutDataTypeStr=Inherit: Same as input  ParamDataTypeStr=Inherit: Same as input
  W(1,2)=wr : Assignment  NumberOfDimensions=2  IndexOptions=Index vector (dialog),Index vector (dialog)  Indices=1,2  OutputSizes=1,1
  W(2,1)=-wr : Assignment  NumberOfDimensions=2  IndexOptions=Index vector (dialog),Index vector (dialog)  Indices=2,1  OutputSizes=1,1
  u1 : Constant  Value=zeros(SMRD.nState,SMRD.nState)
  "[W]" : Outport  VectorParamsAs1DForOutWhenUnconnected=off
  wires:
  u1/1 -> W(1,2)=wr/1
  Gain1/1 -> W(2,1)=-wr/2
  W(1,2)=wr/1 -> W(2,1)=-wr/1
  wr/1 -> W(1,2)=wr/2, Gain1/1
  W(2,1)=-wr/1 -> Gain2/1
  Gain2/1 -> "[W]"/1

== system DQN_Machines/#BACKUP/DQN_Mac_V2_untested/Mechanical model ==
  note: *
  note: Computation of Rotor angle dthetae uses Forward Euler
      | integrator to ensure better accuracy and initialisation.
  note: *
  Te : Inport  PortDimensions=1
  Pm : Inport  Port=2
  1 ----- 2H : Gain  Gain=1/(2*SMRD.H)  SaturateOnIntegerOverflow=on  OutDataTypeStr=Inherit: Same as input  ParamDataTypeStr=Inherit: Same as input
  1_Pb : Gain  Gain=1/SMRD.Pb  SaturateOnIntegerOverflow=on  OutDataTypeStr=Inherit: Same as input  ParamDataTypeStr=Inherit: Same as input
  Delay Prediction : Subsystem
  Digital Clock : DigitalClock  SampleTime=Ts
  F : Gain  Gain=SMRD.F  SaturateOnIntegerOverflow=on  OutDataTypeStr=Inherit: Same as input  ParamDataTypeStr=Inherit: Same as input
  Mux1 : Mux  Inputs=2
  Rate Transition1 : RateTransition  Deterministic=off  OutPortSampleTime=Ts
  Rotor angle dthetae : DiscreteIntegrator  InitialCondition=SMRD.tho  SampleTime=SMRD.Ts  ICPrevOutput=DiscIntNeverNeededParam  ICPrevScaledInput=DiscIntNeverNeededParam
  Rotor speed deviation (dw) : DiscreteIntegrator  IntegratorMethod=Integration: Trapezoidal  InitialCondition=SMRD.dwo  SampleTime=SMRD.Ts  ICPrevOutput=DiscIntNeverNeededParam  ICPrevScaledInput=DiscIntNeverNeededParam
  Sum : Sum  InputSameDT=on  SaturateOnIntegerOverflow=on  OutDataTypeStr=Inherit: Same as first input
  Sum2 : Sum  Inputs=+--  InputSameDT=on  SaturateOnIntegerOverflow=on  OutDataTypeStr=Inherit: Same as first input
  Sum3 : Sum  InputSameDT=on  SaturateOnIntegerOverflow=on  OutDataTypeStr=Inherit: Same as first input
  div : Fcn  Expr=u[2]/u[1]
      mask Display: disp('/')
  nominal speed : Constant
  we base : Gain  Gain=SMRD.wn  SaturateOnIntegerOverflow=on  OutDataTypeStr=Inherit: Same as input  ParamDataTypeStr=Inherit: Same as input
  web2 : Gain  Gain=SMRD.wn  SaturateOnIntegerOverflow=on  OutDataTypeStr=Inherit: Same as input  ParamDataTypeStr=Inherit: Same as input
  dtheta_e : Outport  InitialOutput=0  VectorParamsAs1DForOutWhenUnconnected=off
  we : Outport  Port=2  InitialOutput=0  VectorParamsAs1DForOutWhenUnconnected=off
  theta_e : Outport  Port=3  InitialOutput=0  VectorParamsAs1DForOutWhenUnconnected=off
  wires:
  Delay Prediction/1(dw) -> we base/1, Sum/2  "dw"
  Rate Transition1/1 -> 1_Pb/1
  Rotor angle dthetae/1 -> Sum3/1, dtheta_e/1  "d_theta (rad)"
  web2/1 -> Sum3/2
  Digital Clock/1 -> web2/1
  we base/1 -> Rotor angle dthetae/1
  Rotor speed deviation (dw)/1 -> Delay Prediction/1(in)  "dw"
  nominal speed/1 -> Sum/1
  1 ----- 2H/1 -> Rotor speed deviation (dw)/1
  div/1 -> Sum2/1
  Te/1 -> Sum2/2  "Te"
  Mux1/1 -> div/1
  Pm/1 -> Rate Transition1/1  "Pm"
  1_Pb/1 -> Mux1/2
  F/1 -> Sum2/3
  Sum2/1 -> 1 ----- 2H/1
  Sum/1 -> F/1, we/1, Mux1/1  "n"
  Sum3/1 -> theta_e/1

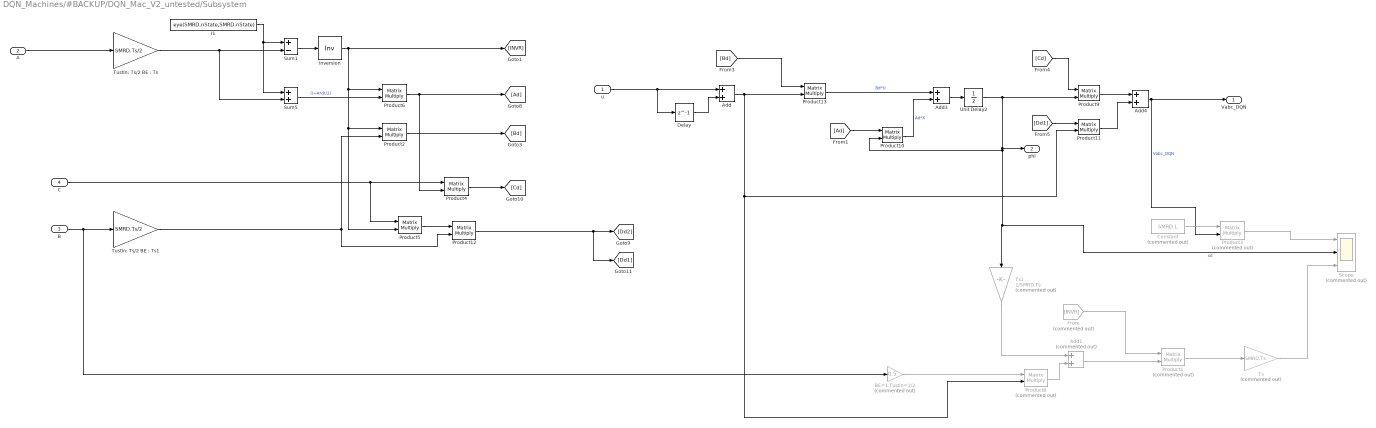
== system DQN_Machines/#BACKUP/DQN_Mac_V2_untested/Subsystem ==
  u : Inport
  A : Inport  Port=2
  B : Inport  Port=3
  C : Inport  Port=4
  Add : Sum
  Add1 : Sum  Commented=on
  Add3 : Sum
  Add4 : Sum
  BE=1 Tustin=1/2 : Gain  Commented=on  Gain=0.5
  Constant : Constant  Commented=on  Value=SMRD.L
  Delay : Delay  DelayLength=1  SampleTime=SMRD.Ts
  From : From  Commented=on  GotoTag=INVR
  I1 : Constant  Value=eye(SMRD.nState,SMRD.nState)
  Product1 : Product  Commented=on  Multiplication=Matrix(*)  SaturateOnIntegerOverflow=on  OutDataTypeStr=Inherit: Same as first input
  Product{2,4..6,9..13} (9 alike) : Product  Multiplication=Matrix(*)  SaturateOnIntegerOverflow=on  OutDataTypeStr=Inherit: Same as first input
  Product3 : Product  Commented=on  Multiplication=Matrix(*)  SaturateOnIntegerOverflow=on  OutDataTypeStr=Inherit: Same as first input
  Product8 : Product  Commented=on  Multiplication=Matrix(*)  SaturateOnIntegerOverflow=on  OutDataTypeStr=Inherit: Same as first input
  Scope : Scope  Commented=on  NumInputPorts=3
  Sum1 : Sum  Inputs=+-  SaturateOnIntegerOverflow=on
  Sum5 : Sum  SaturateOnIntegerOverflow=on
  Ts : Gain  Commented=on  Gain=SMRD.Ts  SaturateOnIntegerOverflow=on  OutDataTypeStr=Inherit: Same as input  ParamDataTypeStr=Inherit: Same as input
  Ts1 : Gain  Commented=on  Gain=1/SMRD.Ts  SaturateOnIntegerOverflow=on  OutDataTypeStr=Inherit: Same as input  ParamDataTypeStr=Inherit: Same as input
  "Tustin: Ts/2 BE : Ts" : Gain  Gain=SMRD.Ts/2  SaturateOnIntegerOverflow=on  OutDataTypeStr=Inherit: Same as input  ParamDataTypeStr=Inherit: Same as input
  "Tustin: Ts/2 BE : Ts1" : Gain  Gain=SMRD.Ts/2  SaturateOnIntegerOverflow=on  OutDataTypeStr=Inherit: Same as input  ParamDataTypeStr=Inherit: Same as input
  Unit Delay2 : UnitDelay  InitialCondition=SMRD.phidq0(1:SMRD.nState)  SampleTime=SMRD.Ts  HasFrameUpgradeWarning=on
  inversion : Product  Inputs=/  Multiplication=Matrix(*)  RndMeth=Zero
  Vabc_DQN : Outport
  phi : Outport  Port=2  VectorParamsAs1DForOutWhenUnconnected=off
  wires:
  Add/1 -> Product8/2, Product11/2, Product13/2
  Product6/1 -> Product4/2, [Ad]
  I1/1 -> Sum5/1, Sum1/1
  "Tustin: Ts/2 BE : Ts1"/1 -> Product12/2, Product2/2
  Product5/1 -> Product12/1
  "Tustin: Ts/2 BE : Ts"/1 -> Sum1/2, Sum5/2
  C/1 -> Product5/1, Product4/1
  Product12/1 -> [Dd1], [Dd2]
  Product11/1 -> Add4/2
  Product10/1 -> Add3/2  "Ad*X"
  [Bd] -> Product13/1
  [Ad] -> Product10/1
  Product4/1 -> [Cd]
  [Dd1] -> Product11/1
  Sum1/1 -> inversion/1
  Sum5/1 -> Product6/2  "(I+A*dt/2)"
  inversion/1 -> [INVR], Product5/2, Product2/1, Product6/1
  Product2/1 -> [Bd]
  [Cd] -> Product9/1
  Product13/1 -> Add3/1  "Bd*U"
  Add3/1 -> Unit Delay2/1
  Product9/1 -> Add4/1
  A/1 -> "Tustin: Ts/2 BE : Ts"/1
  Add4/1 -> Product3/2, Vabc_DQN/1  "Vabc_DQN"
  Add1/1 -> Product1/2
  Product1/1 -> Ts/1
  Product8/1 -> Add1/2
  From/1 -> Product1/1
  B/1 -> BE=1 Tustin=1/2/1, "Tustin: Ts/2 BE : Ts1"/1
  BE=1 Tustin=1/2/1 -> Product8/1
  Unit Delay2/1 -> Scope/2, Ts1/1, Product10/2, phi/1, Product9/2  "xd"
  Ts/1 -> Scope/3
  Ts1/1 -> Add1/1
  u/1 -> Add/1, Delay/1
  Delay/1 -> Add/2
  Constant/1 -> Product3/1
  Product3/1 -> Scope/1

== system DQN_Machines/#BACKUP/DQN_Mac_V3/ABsel2 ==
  v : Inport
  Demux : Demux  Outputs=2
  Mux : Mux  Inputs=3
  Subtract : Sum  Inputs=--
  I : Outport
  wires:
  v/1 -> Demux/1
  Mux/1 -> I/1
  Demux/1 -> Subtract/1, Mux/1
  Demux/2 -> Subtract/2, Mux/2
  Subtract/1 -> Mux/3

== system DQN_Machines/#BACKUP/DQN_Mac_V3/ABsel3 ==
  v : Inport
  Demux : Demux  Outputs=3
  Mux : Mux  Inputs=2
  Subtract : Sum  Inputs=+-
  Subtract1 : Sum  Inputs=+-
  Out1 : Outport
  wires:
  v/1 -> Demux/1
  Mux/1 -> Out1/1
  Demux/1 -> Subtract/1
  Demux/2 -> Subtract1/1, Subtract/2
  Subtract/1 -> Mux/1
  Subtract1/1 -> Mux/2
  Demux/3 -> Subtract1/2

== system DQN_Machines/#BACKUP/DQN_Mac_V3/Discretize BE or Tustin ==
  note: Implement discretized state-space model using Tustin or TBE method
      |
      | BE      -> SM.DSSmethod=1
      | Tustin  -> SM.DSSmethod=2
      |
      |
      | Tustin
      | ------
      | Ad = inv(I - Ts/2*A)*(I + Ts/2*A)
      | Bd = inv(I - Ts/2*A)*B
      | Cd = C*inv(I - Ts/2*A)*Ts
      | Dd = C*inv(I - Ts/2*A)*B*Ts/2  + D  =  Cd*B/2
      |
      | TBE
      | ---
      | Ad = inv(I - Ts*A)
      | Bd = inv(I - Ts*A)*B
      | Cd = C*inv(I - Ts*A)*Ts
      | Dd = C*inv(I - Ts*A)*B*Ts  + D  =  Cd*B
      |
      | I = eye(SM.nState,SM.nState)
  A : Inport
  B : Inport  Port=2
  C : Inport  Port=3
  SW : Inport  Port=4
  Constant6 : Constant  Value=SMRD.Linv
  Gain : Gain  Gain=-1
  I : Constant  Value=eye(SMRD.nState,SMRD.nState)
  Product1 : Product  Multiplication=Matrix(*)  SaturateOnIntegerOverflow=on  OutDataTypeStr=Inherit: Same as first input
  Product2 : Product  Commented=on  Multiplication=Matrix(*)  SaturateOnIntegerOverflow=on  OutDataTypeStr=Inherit: Same as first input
  Product3 : Product  Multiplication=Matrix(*)  SaturateOnIntegerOverflow=on  OutDataTypeStr=Inherit: Same as first input
  Product4 : Product  Multiplication=Matrix(*)  SaturateOnIntegerOverflow=on  OutDataTypeStr=Inherit: Same as first input
  Sum1 : Sum  Inputs=+-  SaturateOnIntegerOverflow=on
  Sum5 : Sum  SaturateOnIntegerOverflow=on
  Switch2 : Switch  Criteria=u2 > Threshold  Threshold=0.5  SaturateOnIntegerOverflow=off  InputSameDT=off
  "Tustin: 1/2 BE : 1.0" : Gain  Gain=1/2  SaturateOnIntegerOverflow=on  OutDataTypeStr=Inherit: Same as input  ParamDataTypeStr=Inherit: Same as input
  "Tustin: Ts/2 BE : Ts" : Gain  Gain=SMRD.Ts/2  SaturateOnIntegerOverflow=on  OutDataTypeStr=Inherit: Same as input  ParamDataTypeStr=Inherit: Same as input
  inversion : Product  Inputs=/  Multiplication=Matrix(*)  RndMeth=Zero
  wbase3 : Gain  Gain=Ts  SaturateOnIntegerOverflow=on  OutDataTypeStr=Inherit: Same as input  ParamDataTypeStr=Inherit: Same as input
  Ad : Outport  VectorParamsAs1DForOutWhenUnconnected=off
  Bd : Outport  Port=2  VectorParamsAs1DForOutWhenUnconnected=off
  Cd : Outport  Port=3  VectorParamsAs1DForOutWhenUnconnected=off
  Dd : Outport  Port=4  VectorParamsAs1DForOutWhenUnconnected=off
  inv(I_Ts/2*A) : Outport  Port=5  VectorParamsAs1DForOutWhenUnconnected=off
  wires:
  "Tustin: Ts/2 BE : Ts"/1 -> Sum1/2, Sum5/2
  Product4/1 -> Ad/1
  A/1 -> "Tustin: Ts/2 BE : Ts"/1
  I/1 -> Sum5/1, Sum1/1
  Sum1/1 -> inversion/1
  inversion/1 -> Product2/2, Product1/1, Product4/1, inv(I_Ts/2*A)/1
  Sum5/1 -> Product4/2
  Product1/1 -> Bd/1
  B/1 -> Product1/2, Product3/2
  C/1 -> Product2/1
  Product3/1 -> "Tustin: 1/2 BE : 1.0"/1
  "Tustin: 1/2 BE : 1.0"/1 -> Dd/1
  Switch2/1 -> wbase3/1
  Constant6/1 -> Gain/1  "Linv"
  SW/1 -> Switch2/2
  Product2/1 -> Switch2/3
  wbase3/1 -> Cd/1, Product3/1
  Gain/1 -> Switch2/1

== system DQN_Machines/#BACKUP/DQN_Mac_V3/Electromagnetic Torque ==
  note: Te computed from stator fluxes and currents
  note: Te=phids*Iqs - phiqs*Ids
  phiqd : Inport
  iqd : Inport  Port=2
  1-1 : Gain  Gain=[1 -1]
  Mult1 : Product  Inputs=**
  Selector1 : Selector  InputPortWidth=2  IndexOptions=Index vector (dialog)  Indices="[2  1]"  OutputSizes=1
  Selector2 : Selector  InputPortWidth=SMRD.nState  IndexOptions=Index vector (dialog)  Indices=[1 2]  OutputSizes=1
  Selector3 : Selector  InputPortWidth=SMRD.nState  IndexOptions=Index vector (dialog)  Indices=[1 2]  OutputSizes=1
  Sum2 : Sum  Inputs=1  SaturateOnIntegerOverflow=on
  Te : Outport  VectorParamsAs1DForOutWhenUnconnected=off
  wires:
  phiqd/1 -> Selector2/1
  Mult1/1 -> Sum2/1
  iqd/1 -> Selector3/1
  1-1/1 -> Mult1/2  "iqs -ids"
  Selector1/1 -> Mult1/1  "phids phiqs"
  Sum2/1 -> Te/1
  Selector2/1 -> Selector1/1
  Selector3/1 -> 1-1/1

== system DQN_Machines/#BACKUP/DQN_Mac_V3/Ihistory_Flux ==
  u : Inport
  B : Inport  Port=2
  Ad : Inport  Port=3
  Bd : Inport  Port=4
  Cd : Inport  Port=5
  D(:,3) : Inport  Port=6
  inv() : Inport  Port=7
  Add : Sum
  Add1 : Sum
  Add2 : Sum
  BE=1 Tustin=1/2 : Gain  Gain=1/2
  Gain : Gain
  Product{1..2,5..8} (6 alike) : Product  Multiplication=Matrix(*)  SaturateOnIntegerOverflow=on  OutDataTypeStr=Inherit: Same as first input
  Selector4 : Selector  InputPortWidth=SMRD.nState  IndexOptions=Index vector (dialog)  Indices=[1 2]  OutputSizes=1
  Ts : Gain  Gain=Ts  SaturateOnIntegerOverflow=on  OutDataTypeStr=Inherit: Same as input  ParamDataTypeStr=Inherit: Same as input
  Unit Delay : UnitDelay  InitialCondition=SMRD.phidq0/Ts  SampleTime=Ts  HasFrameUpgradeWarning=on
  Vf : Selector  InputPortWidth=SMRD.nState  IndexOptions=Index vector (dialog)  Indices=3  OutputSizes=1
  Ihyst : Outport  VectorParamsAs1DForOutWhenUnconnected=off
  phi : Outport  Port=2  VectorParamsAs1DForOutWhenUnconnected=off
  wires:
  BE=1 Tustin=1/2/1 -> Product8/1
  inv()/1 -> Product6/1
  Cd/1 -> Product2/1
  Ad/1 -> Product5/1
  Add1/1 -> Product6/2
  Product8/1 -> Add1/2
  Product6/1 -> Ts/1
  Product5/1 -> Add/2  "Ad*X"
  Unit Delay/1 -> Product5/2, Add1/1, Product2/2  "xd"
  Add/1 -> Unit Delay/1
  Product1/1 -> Add/1  "Bd*U"
  Product2/1 -> Add2/1
  Add2/1 -> Selector4/1
  Product7/1 -> Add2/2
  Vf/1 -> Product7/2
  D(:,3)/1 -> Product7/1
  u/1 -> Product1/2, Gain/1, Product8/2  "u"
  Bd/1 -> Product1/1  "u"
  B/1 -> BE=1 Tustin=1/2/1  "u"
  Selector4/1 -> Ihyst/1
  Gain/1 -> Vf/1
  Ts/1 -> phi/1

== system DQN_Machines/#BACKUP/DQN_Mac_V3/Matrix W ==
  wr : Inport
  Gain1 : Gain  Gain=-1  SaturateOnIntegerOverflow=on  OutDataTypeStr=Inherit: Same as input  ParamDataTypeStr=Inherit: Same as input
  W(1,2)=wr : Assignment  NumberOfDimensions=2  IndexOptions=Index vector (dialog),Index vector (dialog)  Indices=1,2  OutputSizes=1,1
  W(2,1)=-wr : Assignment  NumberOfDimensions=2  IndexOptions=Index vector (dialog),Index vector (dialog)  Indices=2,1  OutputSizes=1,1
  u1 : Constant  Value=zeros(SMRD.nState,SMRD.nState)
  "[W]" : Outport  VectorParamsAs1DForOutWhenUnconnected=off
  wires:
  u1/1 -> W(1,2)=wr/1
  Gain1/1 -> W(2,1)=-wr/2
  W(1,2)=wr/1 -> W(2,1)=-wr/1
  wr/1 -> W(1,2)=wr/2, Gain1/1
  W(2,1)=-wr/1 -> "[W]"/1

== system DQN_Machines/#BACKUP/DQN_Mac_V3/Mechanical model1 ==
  note: *
  Te : Inport  PortDimensions=1
  input : Inport  Port=2
  1 ----- 2H : Gain  Gain=1/(2*SMRD.H)  SaturateOnIntegerOverflow=on  OutDataTypeStr=Inherit: Same as input  ParamDataTypeStr=Inherit: Same as input
  1_Pb : Gain  Gain=1/SMRD.Pb  SaturateOnIntegerOverflow=on  OutDataTypeStr=Inherit: Same as input  ParamDataTypeStr=Inherit: Same as input
  Delay Prediction : Subsystem
  Digital Clock : DigitalClock  SampleTime=SMRD.Ts
  F : Gain  Gain=SMRD.F  SaturateOnIntegerOverflow=on  OutDataTypeStr=Inherit: Same as input  ParamDataTypeStr=Inherit: Same as input
  Mux1 : Mux  Inputs=2
  Rate Transition1 : RateTransition  Deterministic=off  OutPortSampleTime=Ts
  Rotor angle dthetae : DiscreteIntegrator  InitialCondition=SMRD.tho  SampleTime=SMRD.Ts  ICPrevOutput=DiscIntNeverNeededParam  ICPrevScaledInput=DiscIntNeverNeededParam
  Rotor speed deviation (dw) : DiscreteIntegrator  IntegratorMethod=Integration: Trapezoidal  InitialCondition=SMRD.dwo  SampleTime=SMRD.Ts  ICPrevOutput=DiscIntNeverNeededParam  ICPrevScaledInput=DiscIntNeverNeededParam
  Sum : Sum  InputSameDT=on  SaturateOnIntegerOverflow=on  OutDataTypeStr=Inherit: Same as first input
  Sum2 : Sum  Inputs=+--  InputSameDT=on  SaturateOnIntegerOverflow=on  OutDataTypeStr=Inherit: Same as first input
  Sum3 : Sum  InputSameDT=on  SaturateOnIntegerOverflow=on  OutDataTypeStr=Inherit: Same as first input
  div : Fcn  Expr=u[2]/u[1]
      mask Display: disp('/')
  nominal speed : Constant
  we base : Gain  Gain=SMRD.web  SaturateOnIntegerOverflow=on  OutDataTypeStr=Inherit: Same as input  ParamDataTypeStr=Inherit: Same as input
  web2 : Gain  Gain=SMRD.web  SaturateOnIntegerOverflow=on  OutDataTypeStr=Inherit: Same as input  ParamDataTypeStr=Inherit: Same as input
  dtheta_e : Outport  InitialOutput=0  VectorParamsAs1DForOutWhenUnconnected=off
  theta_e : Outport  Port=2  InitialOutput=0  VectorParamsAs1DForOutWhenUnconnected=off
  we : Outport  Port=3  InitialOutput=0  VectorParamsAs1DForOutWhenUnconnected=off
  wires:
  Delay Prediction/1(dw) -> we base/1, Sum/2  "dw"
  Rate Transition1/1 -> 1_Pb/1
  Rotor angle dthetae/1 -> Sum3/1, dtheta_e/1  "d_theta (rad)"
  web2/1 -> Sum3/2
  Digital Clock/1 -> web2/1
  we base/1 -> Rotor angle dthetae/1
  Rotor speed deviation (dw)/1 -> Delay Prediction/1(in)  "dw"
  nominal speed/1 -> Sum/1
  1 ----- 2H/1 -> Rotor speed deviation (dw)/1
  div/1 -> Sum2/1
  Te/1 -> Sum2/2  "Te"
  Mux1/1 -> div/1
  input/1 -> Rate Transition1/1  "Pm"
  1_Pb/1 -> Mux1/2
  F/1 -> Sum2/3
  Sum2/1 -> 1 ----- 2H/1
  Sum/1 -> F/1, we/1, Mux1/1  "n"
  Sum3/1 -> theta_e/1

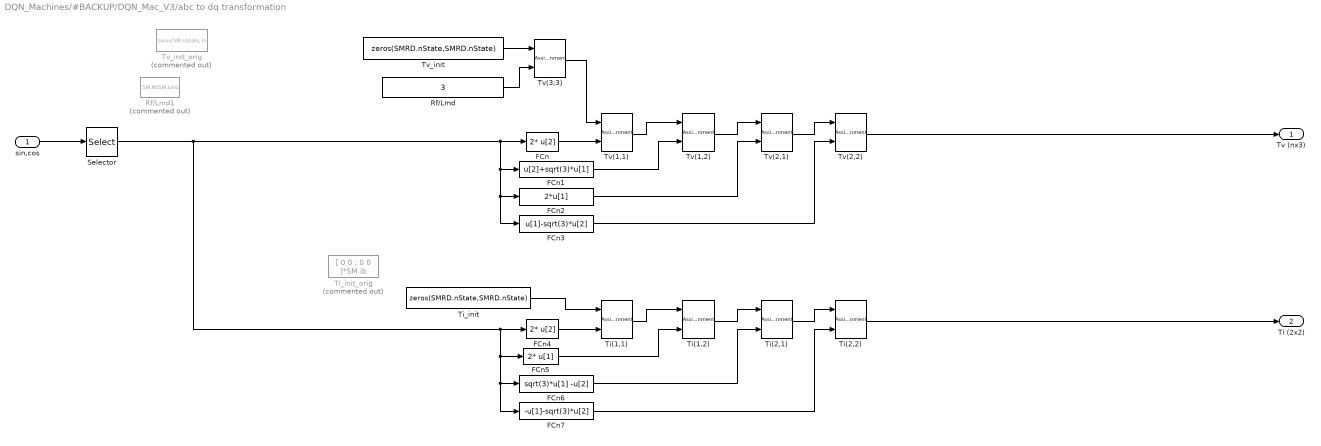
== system DQN_Machines/#BACKUP/DQN_Mac_V3/abc to dq transformation ==
  sin,cos : Inport
  FCn : Fcn  Expr=2* u[2]  SampleTime=Ts
  FCn1 : Fcn  Expr=u[2]+sqrt(3)*u[1]  SampleTime=Ts
  FCn2 : Fcn  Expr=2*u[1]  SampleTime=Ts
  FCn3 : Fcn  Expr=u[1]-sqrt(3)*u[2]  SampleTime=Ts
  FCn4 : Fcn  Expr=2* u[2]  SampleTime=Ts
  FCn5 : Fcn  Expr=2* u[1]  SampleTime=Ts
  FCn6 : Fcn  Expr=sqrt(3)*u[1] -u[2]  SampleTime=Ts
  FCn7 : Fcn  Expr=-u[1]-sqrt(3)*u[2]  SampleTime=Ts
  Rf/Lmd : Constant  Value=3
  Rf/Lmd1 : Constant  Commented=on  Value=SM.Rf/SM.Lmd
  Selector : Selector  InputPortWidth=2  IndexOptions=Index vector (dialog)  Indices=[1 2]  OutputSizes=1
  "Ti(1,1) " : Assignment  NumberOfDimensions=2  DiagnosticForDimensions=Warning  IndexOptions=Index vector (dialog),Index vector (dialog)  Indices=1,1  OutputSizes=1,1
  "Ti(1,2) " : Assignment  NumberOfDimensions=2  DiagnosticForDimensions=Warning  IndexOptions=Index vector (dialog),Index vector (dialog)  Indices=1,2  OutputSizes=1,1
  "Ti(2,1) " : Assignment  NumberOfDimensions=2  DiagnosticForDimensions=Warning  IndexOptions=Index vector (dialog),Index vector (dialog)  Indices=2,1  OutputSizes=1,1
  "Ti(2,2) " : Assignment  NumberOfDimensions=2  DiagnosticForDimensions=Warning  IndexOptions=Index vector (dialog),Index vector (dialog)  Indices=2,2  OutputSizes=1,1
  Ti_init : Constant  Value=zeros(SMRD.nState,SMRD.nState)
  Ti_init_orig : Constant  Commented=on  Value="[ 0  0 ;  0  0  ]*SM.ib"
  Tv(1,1) : Assignment  NumberOfDimensions=2  DiagnosticForDimensions=Warning  IndexOptions=Index vector (dialog),Index vector (dialog)  Indices=1,1  OutputSizes=1,1
  Tv(1,2) : Assignment  NumberOfDimensions=2  DiagnosticForDimensions=Warning  IndexOptions=Index vector (dialog),Index vector (dialog)  Indices=1,2  OutputSizes=1,1
  Tv(2,1) : Assignment  NumberOfDimensions=2  DiagnosticForDimensions=Warning  IndexOptions=Index vector (dialog),Index vector (dialog)  Indices=2,1  OutputSizes=1,1
  Tv(2,2) : Assignment  NumberOfDimensions=2  DiagnosticForDimensions=Warning  IndexOptions=Index vector (dialog),Index vector (dialog)  Indices=2,2  OutputSizes=1,1
  Tv(3,3) : Assignment  NumberOfDimensions=2  DiagnosticForDimensions=Warning  IndexOptions=Index vector (dialog),Index vector (dialog)  Indices=3,3  OutputSizes=1,1
  Tv_init : Constant  Value=zeros(SMRD.nState,SMRD.nState)
  Tv_init_orig : Constant  Commented=on  Value=zeros(SM.nState,3)
  Tv (nx3) : Outport  VectorParamsAs1DForOutWhenUnconnected=off
  Ti (2x2) : Outport  Port=2  VectorParamsAs1DForOutWhenUnconnected=off
  wires:
  Tv(3,3)/1 -> Tv(1,1)/1
  Rf/Lmd/1 -> Tv(3,3)/2
  Tv_init/1 -> Tv(3,3)/1
  FCn7/1 -> "Ti(2,2) "/2
  "Ti(2,1) "/1 -> "Ti(2,2) "/1
  "Ti(1,2) "/1 -> "Ti(2,1) "/1
  FCn6/1 -> "Ti(2,1) "/2
  FCn5/1 -> "Ti(1,2) "/2
  "Ti(1,1) "/1 -> "Ti(1,2) "/1
  FCn4/1 -> "Ti(1,1) "/2
  FCn3/1 -> Tv(2,2)/2
  Tv(2,1)/1 -> Tv(2,2)/1
  Tv(1,2)/1 -> Tv(2,1)/1
  FCn2/1 -> Tv(2,1)/2
  FCn1/1 -> Tv(1,2)/2
  Tv(1,1)/1 -> Tv(1,2)/1
  FCn/1 -> Tv(1,1)/2
  sin,cos/1 -> Selector/1
  Ti_init/1 -> "Ti(1,1) "/1
  Selector/1 -> FCn7/1, FCn6/1, FCn5/1, FCn4/1, FCn/1, FCn1/1, FCn2/1, FCn3/1
  Tv(2,2)/1 -> Tv (nx3)/1
  "Ti(2,2) "/1 -> Ti (2x2)/1
